simulink model "J_tran_idc"  (R2022b)
settings: Solver=VariableStepAuto  StartTime=0.0  StopTime=5.5  FixedStep=.002  RelTol=1e-3
libraries: slpidlib x1
settings Model: Creator=willg  LastModifiedBy=willg

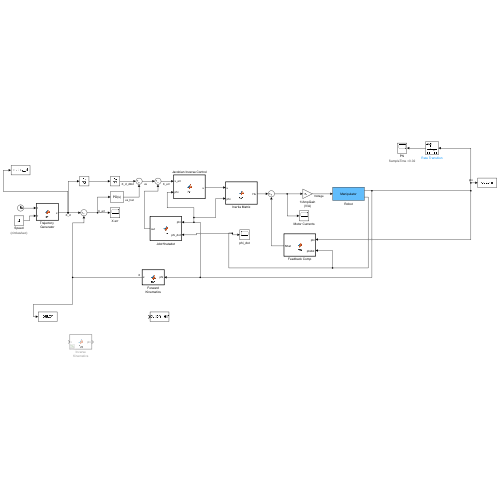
[thumbnail: Simulink's stored preview of the top-level diagram]
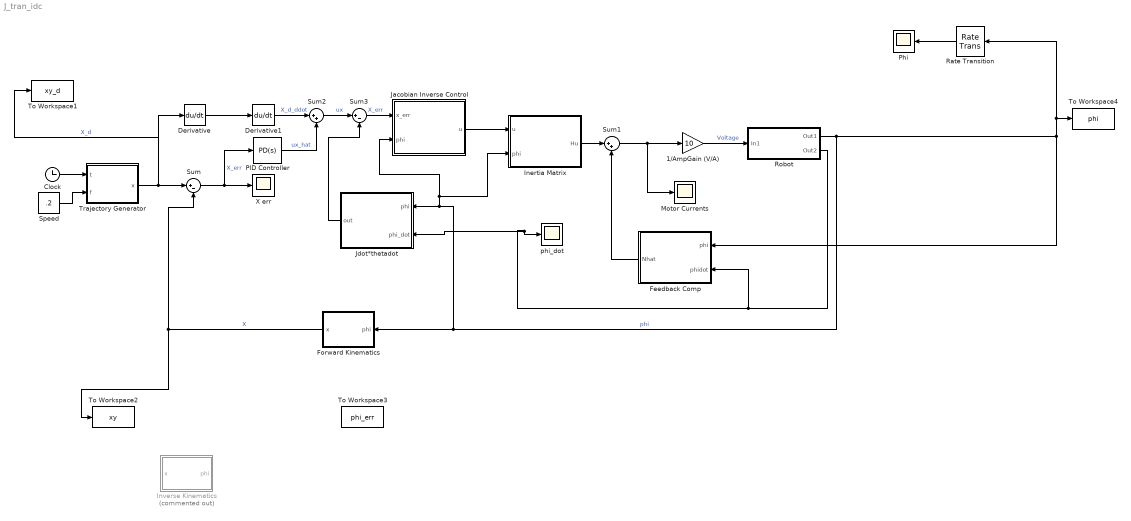
== system J_tran_idc ==
  1/AmpGain (V/A) : Gain  Gain=10
  Clock : Clock
  Derivative : Derivative
  Derivative1 : Derivative
  Feedback Comp : MATLAB Function  TreatAsAtomicUnit=on
  Forward Kinematics : MATLAB Function  TreatAsAtomicUnit=on
  Inertia Matrix : MATLAB Function  TreatAsAtomicUnit=on
  Inverse Kinematics : MATLAB Function  Commented=on  TreatAsAtomicUnit=on
  Jacobian Inverse Control : MATLAB Function  TreatAsAtomicUnit=on
  Jdot*thetadot : MATLAB Function  TreatAsAtomicUnit=on
  Motor Currents : Scope
  PID Controller : slpidlib/PID Controller  Controller=PD  Form=Parallel  TimeDomain=Continuous-time  UseExternalTs=off  SampleTime=-1  IntegratorMethod=Forward Euler  FilterMethod=Forward Euler  ControllerParametersSource=internal  P=1000  I=1  UseKiTs=off  D=50  N=100  UseFilter=on  TunerSelectOption=Transfer Function Based (PID Tuner App)  InitialConditionSource=internal  InitialConditionForIntegrator=0  InitialConditionForFilter=0  DifferentiatorICPrevScaledInput=0  ExternalReset=none  TrackingMode=off  Kt=1  LimitOutput=off  SatLimitsSource=internal  UpperSaturationLimit=inf  LowerSaturationLimit=-inf  LinearizeAsGain=on  AntiWindupMode=none  Kb=1  LimitIntegrator=off  UpperIntegratorSaturationLimit=inf  LowerIntegratorSaturationLimit=-inf  POutMin=[]  POutMax=[]  IOutMin=[]  IOutMax=[]  DOutMin=[]  DOutMax=[]  NOutMin=[]  NOutMax=[]  SumOutMin=[]  SumOutMax=[]  SaturationOutMin=[]  SaturationOutMax=[]  PParamMin=[]  PParamMax=[]  IParamMin=[]  IParamMax=[]  DParamMin=[]  DParamMax=[]  NParamMin=[]  NParamMax=[]  KbParamMin=[]  KbParamMax=[]  KtParamMin=[]  KtParamMax=[]  KbOutMin=[]  KbOutMax=[]  KtOutMin=[]  KtOutMax=[]  IntegratorOutMin=[]  IntegratorOutMax=[]  FilterOutMin=[]  FilterOutMax=[]  SumI1OutMin=[]  SumI1OutMax=[]  SumI2OutMin=[]  SumI2OutMax=[]  SumI3OutMin=[]  SumI3OutMax=[]  SumI4OutMin=[]  SumI4OutMax=[]  SumDOutMin=[]  SumDOutMax=[]  DifferentiatorOutMin=[]  DifferentiatorOutMax=[]  FilterDiffOutCoefMin=[]  FilterDiffOutCoefMax=[]  ReciprocalOutMin=[]  ReciprocalOutMax=[]  SumDenOutMin=[]  SumDenOutMax=[]  SumNumOutMin=[]  SumNumOutMax=[]  DivideOutMin=[]  DivideOutMax=[]  UdiffTsProdOutMin=[]  UdiffTsProdOutMax=[]  NTsProdOutMin=[]  NTsProdOutMax=[]  UintegralTsProdOutMin=[]  UintegralTsProdOutMax=[]  UngainTsProdOutMin=[]  UngainTsProdOutMax=[]  ClampingZeroOutDataTypeStr=Inherit: Inherit via back propagation  ClampingZeroOutMin=[]  ClampingZeroOutMax=[]  FilterDenConstantOutDataTypeStr=Inherit: Inherit via back propagation  FilterDenConstantOutMin=[]  FilterDenConstantOutMax=[]  PCopyOutDataTypeStr=Inherit: Inherit via back propagation  PCopyOutMin=[]  PCopyOutMax=[]  NCopyOutDataTypeStr=Inherit: Inherit via back propagation  NCopyOutMin=[]  NCopyOutMax=[]  IntegratorContinuousStateAttributes=''  IntegratorStateMustResolveToSignalObject=off  IntegratorRTWStateStorageClass=Auto  FilterContinuousStateAttributes=''  FilterStateMustResolveToSignalObject=off  FilterRTWStateStorageClass=Auto  ParallelPVariant=InternalParameters  IdealPVariant=Disabled  IVariant=Disabled  DVariant=InternalParameters  IntegratorVariant=Disabled  SatVariant=Disabled  AWVariant=Disabled  PCopyVariant=Disabled  TRVariant=Disabled  FdbkBlocksVariant=Forward  IdealPFdbkVariant=Disabled  SatFdbkVariant=Disabled  DerivativeFilterVariant=ContFilter  NVariant=InternalParameters  NCopyVariant=Disabled  FilterICVariant=InternalICsFilter  IntegratorICVariant=Disabled  ExternalResetVariant=Disabled  TRSumVariant=Passthrough  SumFdbkVariant=Disabled  SumVariant=Sum_PD  TsampFilterVariant=InternalTs  TsampNgainVariant=Passthrough  TsampIntegralVariant=Disabled_SignalSpec  ExternalSaturationOutDataTypeStr=Inherit: Same as second input
  Phi : Scope
      settings: AttributesFormatString=SampleTime =%<SampleTime>
  Rate Transition : RateTransition  OutPortSampleTimeOpt=Inherit  OutPortSampleTimeMultiple=10  OutPortSampleTime=0.05
  Robot : Subsystem
      mask Display: disp('Manipulator')
  Speed : Constant  Value=.2
      settings: AttributesFormatString=(circles/sec)
  Sum : Sum  Inputs=|+-
  Sum1 : Sum  Inputs=|++
  Sum2 : Sum  Inputs=|++
  Sum3 : Sum  Inputs=|+-
  To Workspace1 : ToWorkspace  VariableName=xy_d  SampleTime=-1
  To Workspace2 : ToWorkspace  VariableName=xy  SampleTime=-1
  To Workspace3 : ToWorkspace  VariableName=phi_err  SampleTime=-1
  To Workspace4 : ToWorkspace  VariableName=phi  SampleTime=-1
  Trajectory Generator : MATLAB Function  TreatAsAtomicUnit=on
  X err : Scope
  phi_dot : Scope
  wires:
  Rate Transition/1 -> Phi/1
  Clock/1 -> Trajectory Generator/1(t)
  Speed/1 -> Trajectory Generator/2(f)
  Trajectory Generator/1(x) -> Derivative/1, Sum/1, To Workspace1/1  "X_d"
  Sum2/1 -> Sum3/1  "ux"
  Derivative/1 -> Derivative1/1
  Sum/1 -> PID Controller/1, X err/1  "X_err"
  PID Controller/1 -> Sum2/2  "ux_hat"
  Derivative1/1 -> Sum2/1  "X_d_ddot"
  Sum3/1 -> Jacobian Inverse Control/1(x_err)  "X_err"
  Jacobian Inverse Control/1(u) -> Inertia Matrix/1(u)
  Sum1/1 -> Motor Currents/1, 1/AmpGain (V/A)/1
  Inertia Matrix/1(Hu) -> Sum1/1
  Forward Kinematics/1(x) -> To Workspace2/1, Sum/2  "X"
  1/AmpGain (V/A)/1 -> Robot/1(In1)  "Voltage"
  Robot/1(Out1) -> Rate Transition/1, To Workspace4/1, Feedback Comp/1(phi), Inertia Matrix/2(phi), Jacobian Inverse Control/2(phi), Jdot*thetadot/1(phi), Forward Kinematics/1(phi)  "phi"
  Feedback Comp/1(Nhat) -> Sum1/2
  Robot/2(Out2) -> Feedback Comp/2(phidot), Jdot*thetadot/2(phi_dot), phi_dot/1
  Jdot*thetadot/1(out) -> Sum3/2

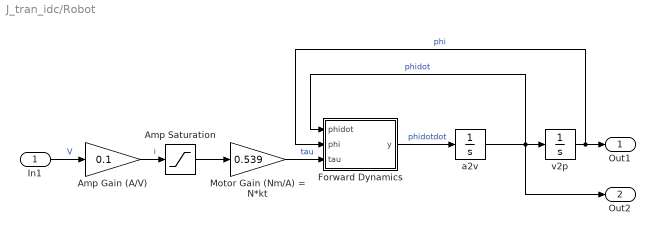
== system J_tran_idc/Robot ==
  In1 : Inport
  Amp Saturation : Saturate  UpperLimit=1  LowerLimit=-1  ZeroCross=off
  Amp Gain (A/V) : Gain  Gain=0.1
  Forward Dynamics : MATLAB Function  TreatAsAtomicUnit=on
  Motor Gain (Nm/A) = N*kt : Gain  Gain=0.539
  a2v : Integrator
  v2p : Integrator  InitialCondition=[1.1934;-0.2661]
  Out1 : Outport
  Out2 : Outport  Port=2
  wires:
  Forward Dynamics/1(y) -> a2v/1  "phidotdot"
  a2v/1 -> v2p/1, Out2/1, Forward Dynamics/1(phidot)  "phidot"
  v2p/1 -> Out1/1, Forward Dynamics/2(phi)  "phi"
  In1/1 -> Amp Gain (A/V)/1  "V"
  Motor Gain (Nm/A) = N*kt/1 -> Forward Dynamics/3(tau)  "tau"
  Amp Saturation/1 -> Motor Gain (Nm/A) = N*kt/1
  Amp Gain (A/V)/1 -> Amp Saturation/1  "i"

== matlab function J_tran_idc/Robot/Forward Dynamics ==
  settings: fimath=|
      | fimath(...
      | 'RoundMode', 'floor',...
      | 'OverflowMode', 'wrap',...
      | 'ProductMode', 'KeepLSB', 'ProductWordLength', 32,...
      | 'SumMode', 'KeepLSB', 'SumWordLength', 32,...
      | 'CastBeforeSum', false)
  data: phidot input double size=2; phi input double size=2; y output double size=2; tau input size=2
function y = fcn(phidot,phi,tau)
% This block supports an embeddable subset of the MATLAB language.
% See the help menu for details. 

a1 = 0.15;  % link 1 length
a2 = 0.15;  % link 2 length
m1 = 0.092;  % link 1 mass  
m2 = 0.077; % link 2 mas
r01 = 0.062; % link 1 center of mass
r12 = 0.036; % link 2 COM
I1 = 0.64e-3;  % link 1 inertia
I2 = 0.30e-3;  % link 2 inertia
Jm1 = 0.65e-6; % motor inertias
Jm2 = 0.65e-6;
b1 = 3.1e-6; % viscous damping constants
b2 = 3.1e-6;
c1 = 0.0001; % coulomb friction constants
c2 = 0.0001;
g = 9.8; % gravitational constant
N1 = 70; % gear ratios
N2 = 70;

H11 = N1^2*Jm1 + I1 + m2*a1^2;
H12 = a1*r12*m2*cos(phi(2)-phi(1));
H21 = H12;
H22 = N2^2*Jm2 + I2;
h = a1*r12*m2*sin(phi(2)-phi(1));
G1 = (r01*m1+a1*m2)*g*cos(phi(1));
G2 = r12*m2*g*cos(phi(2));
F1 = N1^2*b1*phidot(1) + N1*c1*sign(phidot(1));
F2 = N2^2*b2*phidot(2) + N2*c2*sign(phidot(2));

H = [H11 H12; H21 H22]; % inertia matrix
V = [0 -h ;h 0]*[phidot(1)^2;phidot(2)^2]; % centripetal torques
G = [G1;G2]; % gravity torques
F = [F1;F2]; % frictional torques

y = inv(H)*(tau - V - G - F); % y=phidotdot

== matlab function J_tran_idc/Forward Kinematics ==
  settings: fimath=|
      | fimath(...
      | 'RoundMode', 'floor',...
      | 'OverflowMode', 'wrap',...
      | 'ProductMode', 'KeepLSB', 'ProductWordLength', 32,...
      | 'SumMode', 'KeepLSB', 'SumWordLength', 32,...
      | 'CastBeforeSum', false)
  data: x output; phi input
function x = fcn(phi)
% This block supports an embeddable subset of the MATLAB language.
% See the help menu for details. 

a1=0.15;
a2=0.15;
x = [0;0];
x(1) = a1*cos(phi(1))+a2*cos(phi(2));
x(2) = a1*sin(phi(1))+a2*sin(phi(2));

== matlab function J_tran_idc/Inverse Kinematics ==
  settings: fimath=|
      | fimath(...
      | 'RoundMode', 'floor',...
      | 'OverflowMode', 'wrap',...
      | 'ProductMode', 'KeepLSB', 'ProductWordLength', 32,...
      | 'SumMode', 'KeepLSB', 'SumWordLength', 32,...
      | 'CastBeforeSum', false)
  data: x input; phi output
function phi = fcn(x)
% This block supports an embeddable subset of the MATLAB language.
% See the help menu for details. 
a1=0.15;
a2=0.15;
Jt = [1 0;-1 1]; % transmission Jacobian for belt drive

theta = [0;0];
theta(2) = -2*atan(sqrt(((a1+a2)^2-(x(1)^2+x(2)^2))/((x(1)^2+x(2)^2)-(a1-a2)^2)));
theta(1) = atan2(x(2),x(1))-atan2(a2*sin(theta(2)),a1+a2*cos(theta(2)));

phi = inv(Jt)*theta;

== matlab function J_tran_idc/Feedback Comp ==
  settings: fimath=|
      | fimath(...
      | 'RoundMode', 'floor',...
      | 'OverflowMode', 'wrap',...
      | 'ProductMode', 'KeepLSB', 'ProductWordLength', 32,...
      | 'SumMode', 'KeepLSB', 'SumWordLength', 32,...
      | 'CastBeforeSum', false)
  data: Nhat output; phi input; phidot input
function Nhat = fcn(phi, phidot)
% Feedback Comp 

a1 = 0.15;  % link 1 length
a2 = 0.15;  % link 2 length
m1 = 0.092;  % link 1 mass  
m2 = 0.077; % link 2 mas
r01 = 0.062; % link 1 center of mass
r12 = 0.036; % link 2 COM
I1 = 0.64e-3;  % link 1 inertia
I2 = 0.30e-3;  % link 2 inertia
Jm1 = 0.65e-6; % motor inertias
Jm2 = 0.65e-6;
b1 = 3.1e-6; % viscous damping constants
b2 = 3.1e-6;
c1 = 0.0001; % coulomb friction constants
c2 = 0.0001;
g = 9.8; % gravitational constant
N1 = 70; % gear ratios
N2 = 70;

h = a1*r12*m2*sin(phi(2)-phi(1));
G1 = (r01*m1+a1*m2)*g*cos(phi(1));
G2 = r12*m2*g*cos(phi(2));
F1 = N1^2*b1*phidot(1) + N1*c1*sign(phidot(1));
F2 = N2^2*b2*phidot(2) + N2*c2*sign(phidot(2));

V = [0 -h ;h 0]*[phidot(1)^2;phidot(2)^2]; % center torques
G = [G1;G2]; % gravity torques
F = [F1;F2]; % frictional torques

Nhat = V + G + F;

== matlab function J_tran_idc/Trajectory Generator ==
  settings: fimath=|
      | fimath(...
      | 'RoundMode', 'floor',...
      | 'OverflowMode', 'wrap',...
      | 'ProductMode', 'KeepLSB', 'ProductWordLength', 32,...
      | 'SumMode', 'KeepLSB', 'SumWordLength', 32,...
      | 'CastBeforeSum', false)
  data: x output; t input; f input
function x = fcn(t,f)
% This block supports an embeddable subset of the MATLAB language.
% See the help menu for details. 
x = [0;0];

if t<0.5  % accelerate into circling trajectory
    x(1) = 0.075*cos(2*pi*f*t^2) + 0.125;
    x(2) = 0.075*sin(2*pi*f*t^2) + 0.1;
else  % constant speed circling of radius 0.075 about x=[0.125,0.1]
    x(1) = 0.075*cos(2*pi*f*(t-0.25)) + 0.125;
    x(2) = 0.075*sin(2*pi*f*(t-0.25)) + 0.1;
end

== matlab function J_tran_idc/Jdot*thetadot ==
  settings: fimath=|
      | fimath(...
      | 'RoundMode', 'floor',...
      | 'OverflowMode', 'wrap',...
      | 'ProductMode', 'KeepLSB', 'ProductWordLength', 32,...
      | 'SumMode', 'KeepLSB', 'SumWordLength', 32,...
      | 'CastBeforeSum', false)
  data: phi input; out output; phi_dot input
function out = fcn(phi, phi_dot)
% This block supports an embeddable subset of the MATLAB language.
% See the help menu for details. 

a1=0.15;
a2=0.15;
% x = [0;0];
% x(1) = a1*cos(phi(1))+a2*cos(phi(2));
% x(2) = a1*sin(phi(1))+a2*sin(phi(2));

Jt = [1 0;-1 1]; % transmission Jacobian for belt drive

% theta = Jt*phi;
% theta_dot = Jt*phi_dot;

J11 = -a1*cos(phi(1))*phi_dot(1);
J12 = -a2*cos(phi(2))*phi_dot(2);
J21 = a1* -sin(phi(1))*phi_dot(1);
J22 = a2* -sin(phi(2))*phi_dot(2);
J_dot = [J11, J12; J21, J22];

out = J_dot*phi_dot;

== matlab function J_tran_idc/Inertia Matrix ==
  settings: fimath=|
      | fimath(...
      | 'RoundMode', 'floor',...
      | 'OverflowMode', 'wrap',...
      | 'ProductMode', 'KeepLSB', 'ProductWordLength', 32,...
      | 'SumMode', 'KeepLSB', 'SumWordLength', 32,...
      | 'CastBeforeSum', false)
  data: u input; Hu output; phi input
function Hu = fcn(u, phi)
% Inertia Matrix. 

a1 = 0.15;  % link 1 length
a2 = 0.15;  % link 2 length
m1 = 0.092;  % link 1 mass  
m2 = 0.077; % link 2 mas
r01 = 0.062; % link 1 center of mass
r12 = 0.036; % link 2 COM
I1 = 0.64e-3;  % link 1 inertia
I2 = 0.30e-3;  % link 2 inertia
Jm1 = 0.65e-6; % motor inertias
Jm2 = 0.65e-6;
b1 = 3.1e-6; % viscous damping constants
b2 = 3.1e-6;
c1 = 0.0001; % coulomb friction constants
c2 = 0.0001;
g = 9.8; % gravitational constant
N1 = 70; % gear ratios
N2 = 70;

H11 = N1^2*Jm1 + I1 + m2*a1^2;
H12 = a1*r12*m2*cos(phi(2)-phi(1));
H21 = H12;
H22 = N2^2*Jm2 + I2;

H = [H11 H12; H21 H22]; % inertia matrix

Hu = H*u;

== matlab function J_tran_idc/Jacobian Inverse Control ==
  settings: fimath=|
      | fimath(...
      | 'RoundMode', 'floor',...
      | 'OverflowMode', 'wrap',...
      | 'ProductMode', 'KeepLSB', 'ProductWordLength', 32,...
      | 'SumMode', 'KeepLSB', 'SumWordLength', 32,...
      | 'CastBeforeSum', false)
  data: x_err input; u output; phi input
function u = fcn(x_err,phi)
% This block supports an embeddable subset of the MATLAB language.
% See the help menu for details. 

a1=0.15;
a2=0.15;
% x = [0;0];
% x(1) = a1*cos(phi(1))+a2*cos(phi(2));
% x(2) = a1*sin(phi(1))+a2*sin(phi(2));


J11 = -a1*sin(phi(1));
J12 = -a2*sin(phi(2));
J21 = a1*cos(phi(1));
J22 = a2*cos(phi(2));

J = [J11, J12; J21, J22];
u = inv(J)*x_err;
